simulink model "modello_giunto"  (R2025a)
settings: Solver=ode4  StartTime=0.0  StopTime=10.0  FixedStep=0.001  RelTol=1e-3
values from neighbouring files (symbols this model uses):
  K = 1000    [stima_fdt_frequenza.m]
  M = 2    [stima_fdt_frequenza.m]
  Mm = 1    [stima_fdt_frequenza.m]
settings Model: Creator=hp  LastModifiedBy=riccardodaguanno
settings DataIOCC: SaveFormat=StructureWithTime  SaveOutput=off

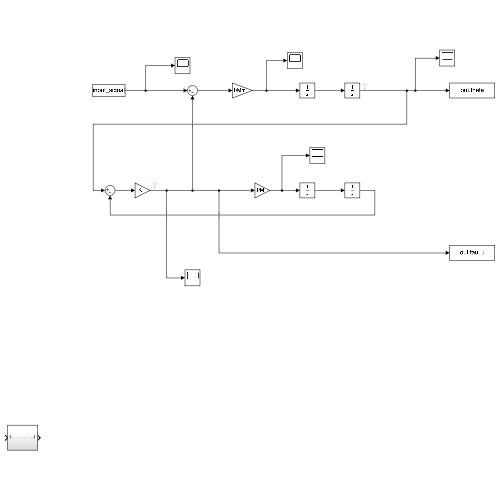
[thumbnail: Simulink's stored preview of the top-level diagram]
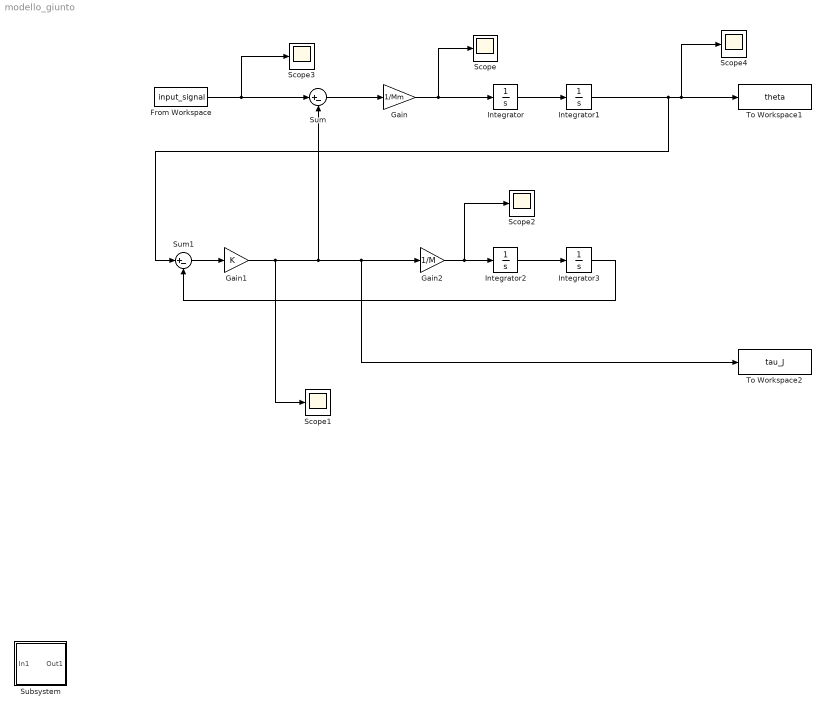
== system modello_giunto ==
  From Workspace : FromWorkspace  VariableName=input_signal
  Gain : Gain  Gain=1/Mm
  Gain1 : Gain  Gain=K
  Gain2 : Gain  Gain=1/M
  Integrator{,1..3} (4 alike) : Integrator
  Scope{,1..4} (5 alike) : Scope
      Scope settings: ActiveDisplayYMinimum=-210.06821527598237  ActiveDisplayYMaximum=210.08656239797062
      Scope1 settings: ActiveDisplayYMinimum=-5.65054  ActiveDisplayYMaximum=6.14623
      Scope2 settings: ActiveDisplayYMinimum=-49.489393224996746  ActiveDisplayYMaximum=61.586816471340484  DataLoggingVariableName=ScopeData2
      Scope3 settings: ActiveDisplayYMinimum=-22.455526242596633  ActiveDisplayYMaximum=34.766035655845286  DataLoggingVariableName=ScopeData3
      Scope4 settings: ActiveDisplayYMinimum=-0.020419427171681381  ActiveDisplayYMaximum=0.48011022910039286  DataLoggingVariableName=ScopeData4
  Subsystem : Subsystem
  Sum : Sum  Inputs=|+-
  Sum1 : Sum  Inputs=|+-
  To Workspace1 : ToWorkspace  VariableName=theta  SaveFormat=Timeseries  SampleTime=-1
  To Workspace2 : ToWorkspace  VariableName=tau_J  SaveFormat=Timeseries  SampleTime=-1
  wires:
  Sum/1 -> Gain/1
  Gain/1 -> Integrator/1, Scope/1
  Integrator/1 -> Integrator1/1
  Integrator1/1 -> Sum1/1, Scope4/1, To Workspace1/1
  Sum1/1 -> Gain1/1
  Gain1/1 -> Scope1/1, To Workspace2/1, Gain2/1, Sum/2
  Gain2/1 -> Scope2/1, Integrator2/1
  Integrator2/1 -> Integrator3/1
  Integrator3/1 -> Sum1/2
  From Workspace/1 -> Scope3/1, Sum/1

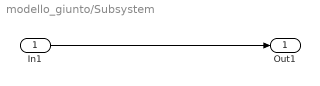
== system modello_giunto/Subsystem ==
  In1 : Inport
  Out1 : Outport
  wires:
  In1/1 -> Out1/1
